simulink model "warehousemultirobot_main_m2020a"  (R2021b)
settings: Solver=VariableStepAuto  StartTime=0.0  StopTime=10000  RelTol=1e-3
model workspace (MAT data in the model file):
  currentR = Simulink.Parameter
  currentR.DataType = 'auto'
  currentR.Complexity = 'real'
  currentR.Dimensions = [0 0]
undefined symbols (not defined in the file or in its folder): chargingStations, loadingStations, packages, rbtprms, shelvesLocations
libraries: mobileRoboticsLib x11, rllib x5, robotmobilelib x5
settings Model: Creator=yekin  LastModifiedBy=yekin
settings SolverCC: AlgebraicLoopSolver=TrustRegion

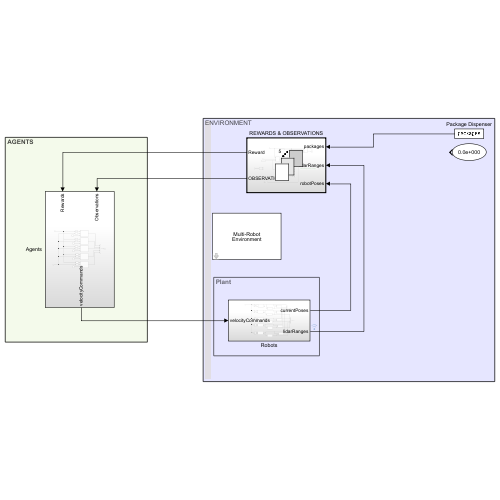
[thumbnail: Simulink's stored preview of the top-level diagram]
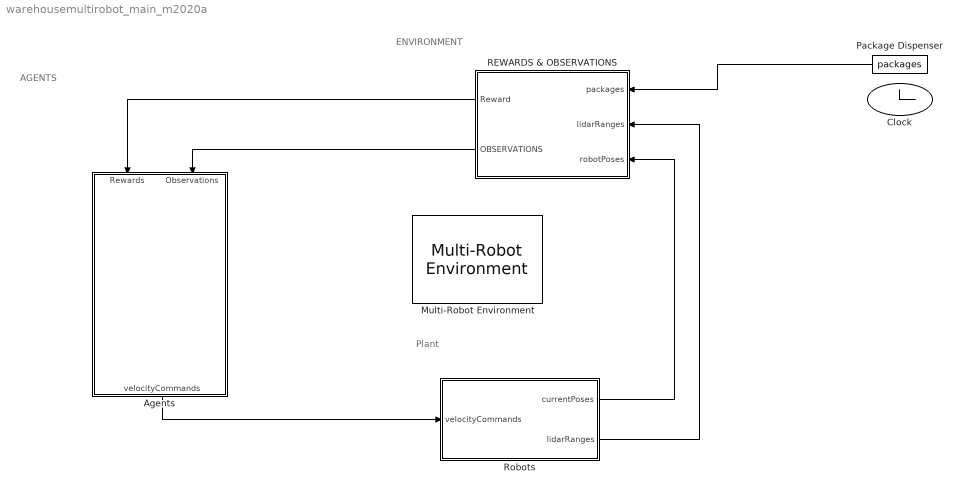
== system warehousemultirobot_main_m2020a ==
  note: ENVIRONMENT
  note: AGENTS
  note: Plant
  Agents : Subsystem
  Clock : Clock
  Multi-Robot Environment : mobileRoboticsLib/Environments/Multi-Robot Environment  numRobots=rbtprms.nums  mapName=map  showWaypoints=off  showObjects=off  objectColors=[ 1, 0, 0; 0, 1, 0; 0, 0, 1 ]  objectMarkers='s'  showRobotIds=on  plotSensorLines=on
      settings: SourceProductName=Mobile Robotics Simulation Toolbox
  Package Dispenser : Constant  Value=packages
  REWARDS & OBSERVATIONS : Subsystem
  Robots : Subsystem
  wires:
  REWARDS & OBSERVATIONS/1(Reward) -> Agents/1(Rewards)
  Package Dispenser/1 -> REWARDS & OBSERVATIONS/1(packages)
  REWARDS & OBSERVATIONS/2(OBSERVATIONS) -> Agents/2(Observations)
  Robots/1(currentPoses) -> REWARDS & OBSERVATIONS/3(robotPoses)
  Robots/2(lidarRanges) -> REWARDS & OBSERVATIONS/2(lidarRanges)
  Agents/1(velocityCommands) -> Robots/1(velocityCommands)

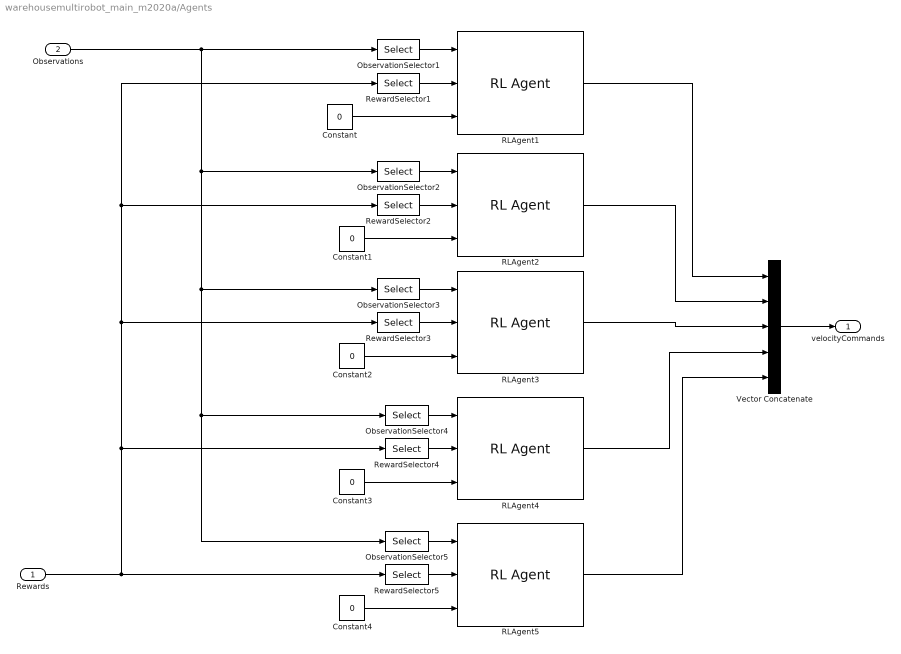
== system warehousemultirobot_main_m2020a/Agents ==
  Rewards : Inport
  Observations : Inport  Port=2
  Constant{,1..4} (5 alike) : Constant  Value=0
  ObservationSelector1 : Selector  NumberOfDimensions=2  InputPortWidth=2  IndexOptions=Select all,Index vector (dialog)  Indices=1,1  OutputSizes=1,1
  ObservationSelector2 : Selector  NumberOfDimensions=2  InputPortWidth=2  IndexOptions=Select all,Index vector (dialog)  Indices=1,2  OutputSizes=1,1
  ObservationSelector3 : Selector  NumberOfDimensions=2  InputPortWidth=2  IndexOptions=Select all,Index vector (dialog)  Indices=1,3  OutputSizes=1,1
  ObservationSelector4 : Selector  NumberOfDimensions=2  InputPortWidth=2  IndexOptions=Select all,Index vector (dialog)  Indices=1,4  OutputSizes=1,1
  ObservationSelector5 : Selector  NumberOfDimensions=2  InputPortWidth=2  IndexOptions=Select all,Index vector (dialog)  Indices=1,5  OutputSizes=1,1
  RLAgent1 : rllib/RL Agent  Agent=agentObj1  ExternalActionAsInput=off  ProvideCumRwd=off  TreatAsDirectFeedthrough=on
  RLAgent2 : rllib/RL Agent  Agent=agentObj2  ExternalActionAsInput=off  ProvideCumRwd=off  TreatAsDirectFeedthrough=on
  RLAgent3 : rllib/RL Agent  Agent=agentObj3  ExternalActionAsInput=off  ProvideCumRwd=off  TreatAsDirectFeedthrough=on
  RLAgent4 : rllib/RL Agent  Agent=agentObj4  ExternalActionAsInput=off  ProvideCumRwd=off  TreatAsDirectFeedthrough=on
  RLAgent5 : rllib/RL Agent  Agent=agentObj5  ExternalActionAsInput=off  ProvideCumRwd=off  TreatAsDirectFeedthrough=on
  RewardSelector1 : Selector  NumberOfDimensions=2  InputPortWidth=2  IndexOptions=Index vector (dialog),Index vector (dialog)  Indices=1,1  OutputSizes=1,1
  RewardSelector2 : Selector  NumberOfDimensions=2  InputPortWidth=2  IndexOptions=Index vector (dialog),Index vector (dialog)  Indices=1,2  OutputSizes=1,1
  RewardSelector3 : Selector  NumberOfDimensions=2  InputPortWidth=2  IndexOptions=Index vector (dialog),Index vector (dialog)  Indices=1,3  OutputSizes=1,1
  RewardSelector4 : Selector  NumberOfDimensions=2  InputPortWidth=2  IndexOptions=Index vector (dialog),Index vector (dialog)  Indices=1,4  OutputSizes=1,1
  RewardSelector5 : Selector  NumberOfDimensions=2  InputPortWidth=2  IndexOptions=Index vector (dialog),Index vector (dialog)  Indices=1,5  OutputSizes=1,1
  Vector Concatenate : Concatenate  NumInputs=5  Mode=Multidimensional array  ConcatenateDimension=2
  velocityCommands : Outport
  wires:
  ObservationSelector5/1 -> RLAgent5/1
  ObservationSelector4/1 -> RLAgent4/1
  ObservationSelector3/1 -> RLAgent3/1
  ObservationSelector2/1 -> RLAgent2/1
  ObservationSelector1/1 -> RLAgent1/1
  RewardSelector5/1 -> RLAgent5/2
  RewardSelector4/1 -> RLAgent4/2
  RewardSelector3/1 -> RLAgent3/2
  RewardSelector2/1 -> RLAgent2/2
  RewardSelector1/1 -> RLAgent1/2
  Observations/1 -> ObservationSelector4/1, ObservationSelector5/1, ObservationSelector3/1, ObservationSelector2/1, ObservationSelector1/1
  Rewards/1 -> RewardSelector2/1, RewardSelector1/1, RewardSelector3/1, RewardSelector4/1, RewardSelector5/1
  Vector Concatenate/1 -> velocityCommands/1
  RLAgent1/1 -> Vector Concatenate/1
  RLAgent2/1 -> Vector Concatenate/2
  RLAgent3/1 -> Vector Concatenate/3
  RLAgent4/1 -> Vector Concatenate/4
  RLAgent5/1 -> Vector Concatenate/5
  Constant/1 -> RLAgent1/3
  Constant4/1 -> RLAgent5/3
  Constant3/1 -> RLAgent4/3
  Constant2/1 -> RLAgent3/3
  Constant1/1 -> RLAgent2/3

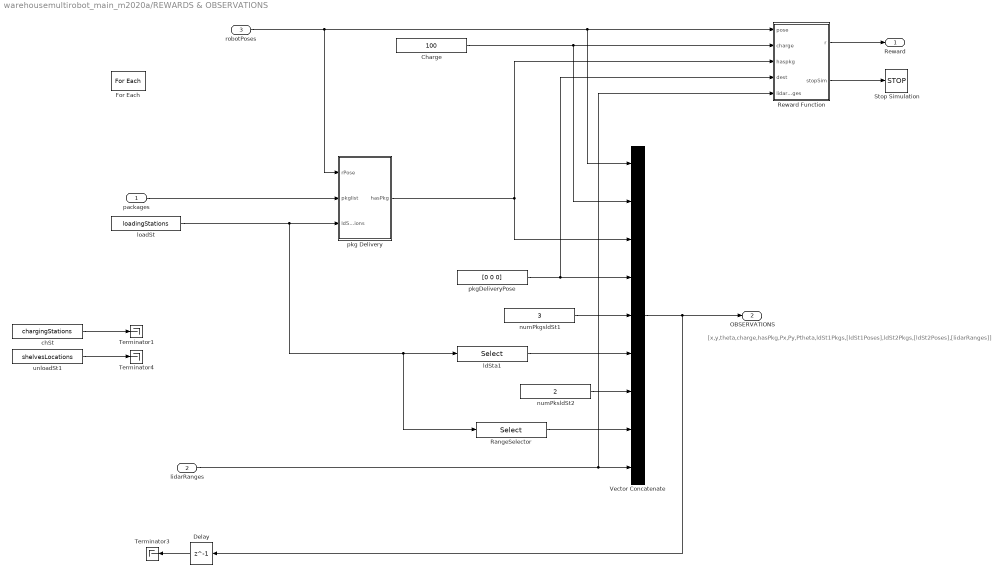
== system warehousemultirobot_main_m2020a/REWARDS & OBSERVATIONS ==
  note: [x,y,theta,charge,hasPkg,Px,Py,Ptheta,ldSt1Pkgs,[ldSt1Poses],ldSt2Pkgs,[ldSt2Poses],[lidarRanges]]
  packages : Inport
  lidarRanges : Inport  Port=2  Partition=on  PartitionDimension=2  PartitionWidth=1  PartitionOffset=0
  robotPoses : Inport  Port=3  Partition=on  PartitionDimension=2  PartitionWidth=1  PartitionOffset=0
  Charge : Constant  Value=100
  Delay : Delay  DelayLength=1
  For Each : ForEach  DisableCoverage=on
  RangeSelector : Selector  NumberOfDimensions=2  InputPortWidth=12  IndexOptions=Select all,Index vector (dialog)  Indices=1,2  OutputSizes=1,1
  Reward Function : MATLAB Function  TreatAsAtomicUnit=on
  Stop Simulation : Stop
  Terminator1 : Terminator
  Terminator3 : Terminator
  Terminator4 : Terminator
  Vector Concatenate : Concatenate  NumInputs=9  Mode=Multidimensional array
  chSt : Constant  Value=chargingStations
  ldSta1 : Selector  NumberOfDimensions=2  InputPortWidth=12  IndexOptions=Select all,Index vector (dialog)  Indices=1,1  OutputSizes=1,1
  loadSt : Constant  Value=loadingStations
  numPkgsldSt1 : Constant  Value=3
  numPksldSt2 : Constant  Value=2
  pkg Delivery : MATLAB Function  TreatAsAtomicUnit=on
  pkgDeliveryPose : Constant  Value=[0 0 0]
  unloadSt1 : Constant  Value=shelvesLocations
  Reward : Outport  ConcatenationDimension=2
  OBSERVATIONS : Outport  Port=2  ConcatenationDimension=2
  wires:
  packages/1 -> pkg Delivery/2(pkglist)
  chSt/1 -> Terminator1/1
  unloadSt1/1 -> Terminator4/1
  robotPoses/1 -> Vector Concatenate/1, Reward Function/1(pose), pkg Delivery/1(rPose)
  Vector Concatenate/1 -> OBSERVATIONS/1, Delay/1
  Charge/1 -> Vector Concatenate/2, Reward Function/2(charge)
  pkg Delivery/1(hasPkg) -> Reward Function/3(haspkg), Vector Concatenate/3
  pkgDeliveryPose/1 -> Reward Function/4(dest), Vector Concatenate/4
  ldSta1/1 -> Vector Concatenate/6
  numPkgsldSt1/1 -> Vector Concatenate/5
  lidarRanges/1 -> Reward Function/5(lidarRanges), Vector Concatenate/9
  loadSt/1 -> RangeSelector/1, ldSta1/1, pkg Delivery/3(ldStations)
  Delay/1 -> Terminator3/1
  Reward Function/1(r) -> Reward/1
  numPksldSt2/1 -> Vector Concatenate/7
  RangeSelector/1 -> Vector Concatenate/8
  Reward Function/2(stopSim) -> Stop Simulation/1

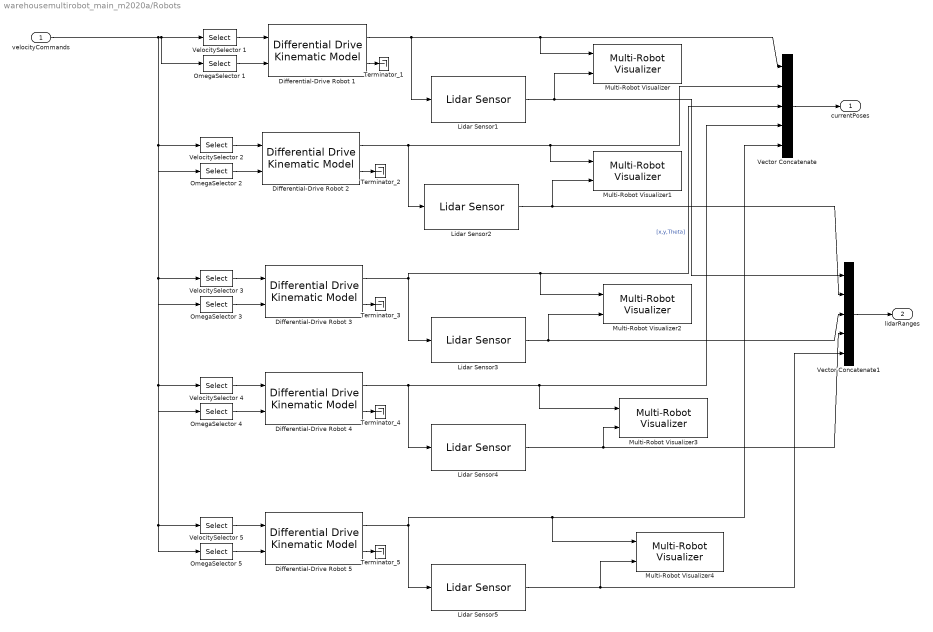
== system warehousemultirobot_main_m2020a/Robots ==
  velocityCommands : Inport
  Differential-Drive Robot 1 : robotmobilelib/Differential Drive Kinematic Model  VehicleInputs=Vehicle Speed & Heading Angular Velocity  WheelRadius=rbtprms.wheelRadius  WheelSpeedRange=[-rbtprms.maxLinSpeed rbtprms.maxLinSpeed]  TrackWidth=rbtprms.trackWidth  InitialState=chargingStations(:,1)  SimulateUsing=Interpreted execution
      settings: SourceProductBaseCode=RO
  Differential-Drive Robot 2 : robotmobilelib/Differential Drive Kinematic Model  VehicleInputs=Vehicle Speed & Heading Angular Velocity  WheelRadius=rbtprms.wheelRadius  WheelSpeedRange=[-rbtprms.maxLinSpeed rbtprms.maxLinSpeed]  TrackWidth=rbtprms.trackWidth  InitialState=chargingStations(:,2)  SimulateUsing=Interpreted execution
      settings: SourceProductBaseCode=RO
  Differential-Drive Robot 3 : robotmobilelib/Differential Drive Kinematic Model  VehicleInputs=Vehicle Speed & Heading Angular Velocity  WheelRadius=rbtprms.wheelRadius  WheelSpeedRange=[-rbtprms.maxLinSpeed rbtprms.maxLinSpeed]  TrackWidth=rbtprms.trackWidth  InitialState=chargingStations(:,3)  SimulateUsing=Interpreted execution
      settings: SourceProductBaseCode=RO
  Differential-Drive Robot 4 : robotmobilelib/Differential Drive Kinematic Model  VehicleInputs=Vehicle Speed & Heading Angular Velocity  WheelRadius=rbtprms.wheelRadius  WheelSpeedRange=[-rbtprms.maxLinSpeed rbtprms.maxLinSpeed]  TrackWidth=rbtprms.trackWidth  InitialState=chargingStations(:,4)  SimulateUsing=Interpreted execution
      settings: SourceProductBaseCode=RO
  Differential-Drive Robot 5 : robotmobilelib/Differential Drive Kinematic Model  VehicleInputs=Vehicle Speed & Heading Angular Velocity  WheelRadius=rbtprms.wheelRadius  WheelSpeedRange=[-rbtprms.maxLinSpeed rbtprms.maxLinSpeed]  TrackWidth=rbtprms.trackWidth  InitialState=chargingStations(:,5)  SimulateUsing=Interpreted execution
      settings: SourceProductBaseCode=RO
  Lidar Sensor{1..5} (5 alike) : mobileRoboticsLib/Environments/Lidar Sensor  mapName=map  sensorOffset=[ 0, 0 ]  scanAngles=rbtprms.lidarScnAngles  maxRange=rbtprms.maxLidarRange
      settings: SourceProductName=Mobile Robotics Simulation Toolbox
  Multi-Robot Visualizer : mobileRoboticsLib/Environments/Multi-Robot Visualizer  idx=1  radius=rbtprms.radius  robotColor=[0 0 1]  showTraj=on  hasLidar=on  sensorOffset=[0,0]  scanAngles=rbtprms.lidarScnAngles  maxNumScans=0  hasObjDetector=off  objDetectorOffset=[0,0]  objDetectorAngle=0  objDetectorFOV=pi/3  objDetectorMaxRange=5  hasRobotDetector=off  robotDetectorOffset=[0,0]  robotDetectorAngle=0  robotDetectorFOV=pi/3  robotDetectorMaxRange=5  robotDetectorNumDetections=0
      settings: SourceProductName=Mobile Robotics Simulation Toolbox
  Multi-Robot Visualizer1 : mobileRoboticsLib/Environments/Multi-Robot Visualizer  idx=2  radius=rbtprms.radius  robotColor=[0 1 0]  showTraj=on  hasLidar=on  sensorOffset=[0,0]  scanAngles=rbtprms.lidarScnAngles  maxNumScans=0  hasObjDetector=off  objDetectorOffset=[0,0]  objDetectorAngle=0  objDetectorFOV=pi/3  objDetectorMaxRange=5  hasRobotDetector=off  robotDetectorOffset=[0,0]  robotDetectorAngle=0  robotDetectorFOV=pi/3  robotDetectorMaxRange=5  robotDetectorNumDetections=0
      settings: SourceProductName=Mobile Robotics Simulation Toolbox
  Multi-Robot Visualizer2 : mobileRoboticsLib/Environments/Multi-Robot Visualizer  idx=3  radius=rbtprms.radius  robotColor=[0 1 1]  showTraj=on  hasLidar=on  sensorOffset=[0,0]  scanAngles=rbtprms.lidarScnAngles  maxNumScans=0  hasObjDetector=off  objDetectorOffset=[0,0]  objDetectorAngle=0  objDetectorFOV=pi/3  objDetectorMaxRange=5  hasRobotDetector=off  robotDetectorOffset=[0,0]  robotDetectorAngle=0  robotDetectorFOV=pi/3  robotDetectorMaxRange=5  robotDetectorNumDetections=0
      settings: SourceProductName=Mobile Robotics Simulation Toolbox
  Multi-Robot Visualizer3 : mobileRoboticsLib/Environments/Multi-Robot Visualizer  idx=4  radius=rbtprms.radius  robotColor=[1 0 0]  showTraj=on  hasLidar=on  sensorOffset=[0,0]  scanAngles=rbtprms.lidarScnAngles  maxNumScans=0  hasObjDetector=off  objDetectorOffset=[0,0]  objDetectorAngle=0  objDetectorFOV=pi/3  objDetectorMaxRange=5  hasRobotDetector=off  robotDetectorOffset=[0,0]  robotDetectorAngle=0  robotDetectorFOV=pi/3  robotDetectorMaxRange=5  robotDetectorNumDetections=0
      settings: SourceProductName=Mobile Robotics Simulation Toolbox
  Multi-Robot Visualizer4 : mobileRoboticsLib/Environments/Multi-Robot Visualizer  idx=5  radius=rbtprms.radius  robotColor=[1 0 1]  showTraj=on  hasLidar=on  sensorOffset=[0,0]  scanAngles=rbtprms.lidarScnAngles  maxNumScans=0  hasObjDetector=off  objDetectorOffset=[0,0]  objDetectorAngle=0  objDetectorFOV=pi/3  objDetectorMaxRange=5  hasRobotDetector=off  robotDetectorOffset=[0,0]  robotDetectorAngle=0  robotDetectorFOV=pi/3  robotDetectorMaxRange=5  robotDetectorNumDetections=0
      settings: SourceProductName=Mobile Robotics Simulation Toolbox
  OmegaSelector 1 : Selector  NumberOfDimensions=2  InputPortWidth=2  IndexOptions=Index vector (dialog),Index vector (dialog)  Indices=2,1  OutputSizes=1,1
  OmegaSelector 2 : Selector  NumberOfDimensions=2  InputPortWidth=2  IndexOptions=Index vector (dialog),Index vector (dialog)  Indices=2,2  OutputSizes=1,1
  OmegaSelector 3 : Selector  NumberOfDimensions=2  InputPortWidth=2  IndexOptions=Index vector (dialog),Index vector (dialog)  Indices=2,3  OutputSizes=1,1
  OmegaSelector 4 : Selector  NumberOfDimensions=2  InputPortWidth=2  IndexOptions=Index vector (dialog),Index vector (dialog)  Indices=2,4  OutputSizes=1,1
  OmegaSelector 5 : Selector  NumberOfDimensions=2  InputPortWidth=2  IndexOptions=Index vector (dialog),Index vector (dialog)  Indices=2,5  OutputSizes=1,1
  Terminator_{1..5} (5 alike) : Terminator
  Vector Concatenate : Concatenate  NumInputs=5  Mode=Multidimensional array  ConcatenateDimension=2
  Vector Concatenate1 : Concatenate  NumInputs=5  Mode=Multidimensional array  ConcatenateDimension=2
  VelocitySelector 1 : Selector  NumberOfDimensions=2  InputPortWidth=2  IndexOptions=Index vector (dialog),Index vector (dialog)  Indices=1,1  OutputSizes=1,1
  VelocitySelector 2 : Selector  NumberOfDimensions=2  InputPortWidth=2  IndexOptions=Index vector (dialog),Index vector (dialog)  Indices=1,2  OutputSizes=1,1
  VelocitySelector 3 : Selector  NumberOfDimensions=2  InputPortWidth=2  IndexOptions=Index vector (dialog),Index vector (dialog)  Indices=1,3  OutputSizes=1,1
  VelocitySelector 4 : Selector  NumberOfDimensions=2  InputPortWidth=2  IndexOptions=Index vector (dialog),Index vector (dialog)  Indices=1,4  OutputSizes=1,1
  VelocitySelector 5 : Selector  NumberOfDimensions=2  InputPortWidth=2  IndexOptions=Index vector (dialog),Index vector (dialog)  Indices=1,5  OutputSizes=1,1
  currentPoses : Outport
  lidarRanges : Outport  Port=2
  wires:
  VelocitySelector 1/1 -> Differential-Drive Robot 1/1
  OmegaSelector 1/1 -> Differential-Drive Robot 1/2
  Differential-Drive Robot 1/2 -> Terminator_1/1
  Lidar Sensor1/1 -> Multi-Robot Visualizer/2, Vector Concatenate1/1
  Differential-Drive Robot 1/1 -> Lidar Sensor1/1, Multi-Robot Visualizer/1, Vector Concatenate/1
  Differential-Drive Robot 2/1 -> Lidar Sensor2/1, Multi-Robot Visualizer1/1, Vector Concatenate/2
  OmegaSelector 2/1 -> Differential-Drive Robot 2/2
  VelocitySelector 2/1 -> Differential-Drive Robot 2/1
  Differential-Drive Robot 2/2 -> Terminator_2/1
  Lidar Sensor2/1 -> Multi-Robot Visualizer1/2, Vector Concatenate1/2
  Differential-Drive Robot 3/1 -> Lidar Sensor3/1, Multi-Robot Visualizer2/1, Vector Concatenate/3  "[x,y,Theta]"
  OmegaSelector 3/1 -> Differential-Drive Robot 3/2
  VelocitySelector 3/1 -> Differential-Drive Robot 3/1
  Differential-Drive Robot 3/2 -> Terminator_3/1
  Differential-Drive Robot 4/1 -> Lidar Sensor4/1, Multi-Robot Visualizer3/1, Vector Concatenate/4
  OmegaSelector 4/1 -> Differential-Drive Robot 4/2
  VelocitySelector 4/1 -> Differential-Drive Robot 4/1
  Differential-Drive Robot 4/2 -> Terminator_4/1
  Lidar Sensor4/1 -> Multi-Robot Visualizer3/2, Vector Concatenate1/4
  Differential-Drive Robot 5/1 -> Lidar Sensor5/1, Multi-Robot Visualizer4/1, Vector Concatenate/5
  OmegaSelector 5/1 -> Differential-Drive Robot 5/2
  VelocitySelector 5/1 -> Differential-Drive Robot 5/1
  Differential-Drive Robot 5/2 -> Terminator_5/1
  velocityCommands/1 -> VelocitySelector 5/1, OmegaSelector 5/1, VelocitySelector 4/1, OmegaSelector 4/1, VelocitySelector 3/1, OmegaSelector 3/1, VelocitySelector 2/1, OmegaSelector 2/1, VelocitySelector 1/1, OmegaSelector 1/1
  Lidar Sensor5/1 -> Multi-Robot Visualizer4/2, Vector Concatenate1/5
  Lidar Sensor3/1 -> Multi-Robot Visualizer2/2, Vector Concatenate1/3
  Vector Concatenate1/1 -> lidarRanges/1
  Vector Concatenate/1 -> currentPoses/1

== matlab function warehousemultirobot_main_m2020a/REWARDS & OBSERVATIONS/pkg Delivery ==
  data: rPose input; pkglist input; ldStations input; hasPkg output
function hasPkg = fcn(rPose, pkglist, ldStations)

hasPkg = 0;

== matlab function warehousemultirobot_main_m2020a/REWARDS & OBSERVATIONS/Reward Function ==
  data: pose input; charge input; r output; haspkg input; dest input; lidarRanges input; stopSim output
function [r,stopSim] = fcn(pose, charge, haspkg, dest, lidarRanges)
    r = 0;
    minrange = min(lidarRanges);
    if minrange < 0.5
        stopSim = true;
    else
        stopSim = false;
    end

    if haspkg > 0
        d = norm(pose-dest);
  
        r = (-1/minrange) - d;
    else
        r = (-1/minrange);
    end
